simulink model "LQR"  (R2020a)
settings: Solver=VariableStepAuto  StartTime=0.0  StopTime=30  RelTol=1e-3
values from neighbouring files (symbols this model uses):
  A = [5.13674577679 1 0 0 0 0 -11.4974040302 0 1 0 0 0 ... (36 elements, 6x6)]    [state_space_model.mat]
  B = [1 0 0 0 0 0]    [state_space_model.mat]
  C = [0 -8.56427886647e-05 0.000639852636745 -0.000603207268883 0 0]    [state_space_model.mat]
  Ts = 1/fs    (= 0.01)    [Control_script.m]
undefined symbols (not defined in the file or in its folder): Atrue, Btrue, Ctrue, Dtrue
settings Model: Creator=franc  LastModifiedBy=franc

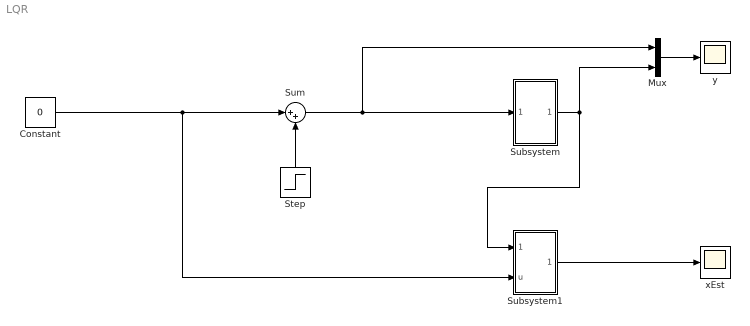
== system LQR ==
  Constant : Constant  Value=0
  Mux : Mux  Inputs=2
  Step : Step  SampleTime=0
  Subsystem : Subsystem
  Subsystem1 : Subsystem
  Sum : Sum  Inputs=|++
  xEst : Scope
  y : Scope
  wires:
  Constant/1 -> Subsystem1/2(u), Sum/1
  Mux/1 -> y/1
  Subsystem/1(y_mod) -> Subsystem1/1(y_mod), Mux/2
  Sum/1 -> Mux/1, Subsystem/1(In1)
  Step/1 -> Sum/2
  Subsystem1/1(x_est) -> xEst/1

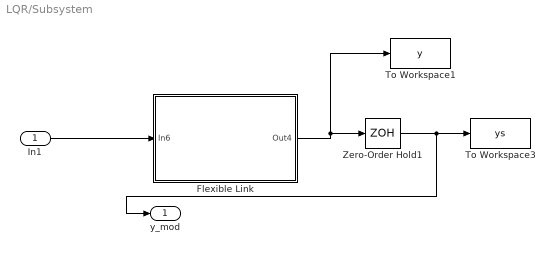
== system LQR/Subsystem ==
  In1 : Inport
  Flexible Link : Subsystem
      mask Display: image('quanserlink.jpg')
  To Workspace1 : ToWorkspace  VariableName=y  SampleTime=-1
  To Workspace3 : ToWorkspace  VariableName=ys  SampleTime=Ts
  Zero-Order Hold1 : ZeroOrderHold  SampleTime=Ts
  y_mod : Outport
  wires:
  Zero-Order Hold1/1 -> y_mod/1, To Workspace3/1
  In1/1 -> Flexible Link/1(In6)
  Flexible Link/1(Out4) -> To Workspace1/1, Zero-Order Hold1/1

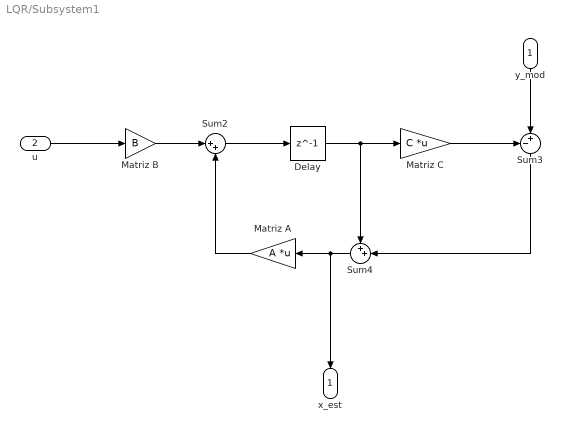
== system LQR/Subsystem1 ==
  y_mod : Inport
  u : Inport  Port=2
  Delay : Delay  DelayLength=1  InitialCondition=0
  Matriz A : Gain  Gain=A  Multiplication=Matrix(K*u)
  Matriz B : Gain  Gain=B
  Matriz C : Gain  Gain=C  Multiplication=Matrix(K*u)
  Sum2 : Sum  Inputs=|++
  Sum3 : Sum  Inputs=-+|
  Sum4 : Sum  Inputs=++|
  x_est : Outport  VectorParamsAs1DForOutWhenUnconnected=off
  wires:
  Sum4/1 -> x_est/1, Matriz A/1
  Sum2/1 -> Delay/1
  Matriz C/1 -> Sum3/1
  u/1 -> Matriz B/1
  Matriz A/1 -> Sum2/2
  Delay/1 -> Sum4/1, Matriz C/1
  Matriz B/1 -> Sum2/1
  y_mod/1 -> Sum3/2
  Sum3/1 -> Sum4/2

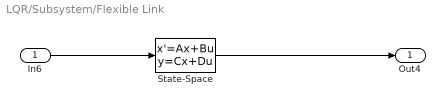
== system LQR/Subsystem/Flexible Link ==
  In6 : Inport
  State-Space : StateSpace  A=Atrue  B=Btrue  C=Ctrue  D=Dtrue  InitialCondition=0
  Out4 : Outport
  wires:
  State-Space/1 -> Out4/1
  In6/1 -> State-Space/1
